simulink model "model"  (R2016a)
settings: Solver=VariableStepAuto  StartTime=0.0  StopTime=30  RelTol=1e-3
values from neighbouring files (symbols this model uses):
  d = 1000    [RobotConstants.mat]
  l0 = 0.16    [RobotConstants.mat]
libraries: simulink x1
settings Model: Creator=Florian  LastModifiedBy=Florian
settings DataIOCC: ExternalInput=[l0]

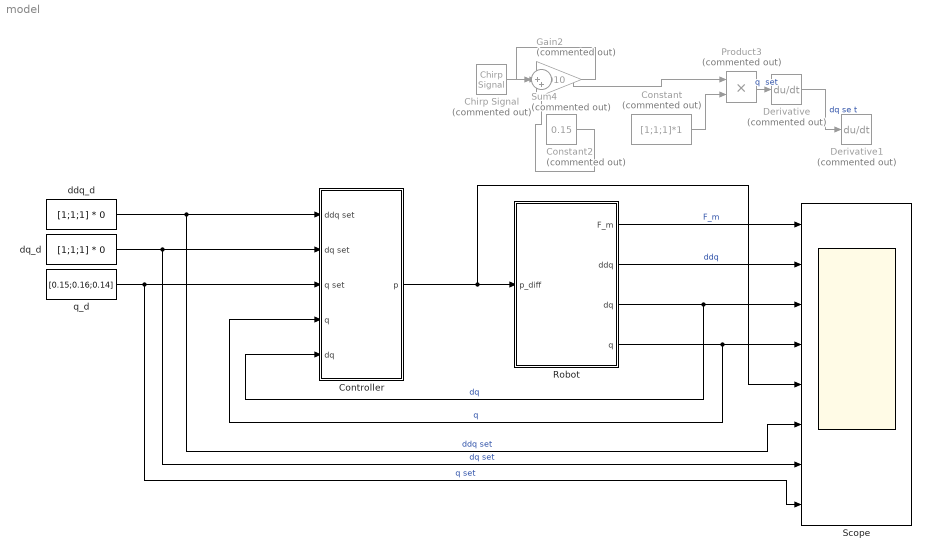
== system model ==
  Chirp Signal : simulink/Sources/Chirp Signal  Commented=on  f1=0.1  T=30  f2=0.1
  Constant : Constant  Commented=on  Value=[1;1;1]*1
  Constant2 : Constant  Commented=on  Value=0.15
  Controller : Subsystem
  Derivative : Derivative  Commented=on
  Derivative1 : Derivative  Commented=on
  Gain2 : Gain  Commented=on  Gain=0.010
  Product3 : Product  Commented=on
  Robot : Subsystem
      mask Display: image('C:\Users\Florian\Documents\Uni\IDP\DVD\Pictures\contibot1seg.JPG');
  Scope : Scope  NumInputPorts=8
  Sum4 : Sum  Commented=on  Inputs=|++
  ddq_d : Constant  Value=[1;1;1] * 0  SampleTime=0.01
  dq_d : Constant  Value=[1;1;1] * 0  SampleTime=0.01
  q_d : Constant  Value=[0.15;0.16;0.14]  SampleTime=0.01
  wires:
  Robot/1(F_m) -> Scope/1  "F_m"
  Robot/2(ddq) -> Scope/2  "ddq"
  Robot/3(dq) -> Controller/5(dq), Scope/3  "dq"
  Robot/4(q) -> Controller/4(q), Scope/4  "q"
  Constant/1 -> Product3/2
  Chirp Signal/1 -> Gain2/1
  Gain2/1 -> Sum4/1
  Sum4/1 -> Product3/1
  Constant2/1 -> Sum4/2
  Product3/1 -> Derivative/1  "q  set"
  Derivative/1 -> Derivative1/1  "dq se t"
  ddq_d/1 -> Controller/1(ddq set), Scope/6  "ddq set"
  Controller/1(p) -> Scope/5, Robot/1(p_diff)
  dq_d/1 -> Scope/7, Controller/2(dq set)  "dq set"
  q_d/1 -> Scope/8, Controller/3(q set)  "q set"

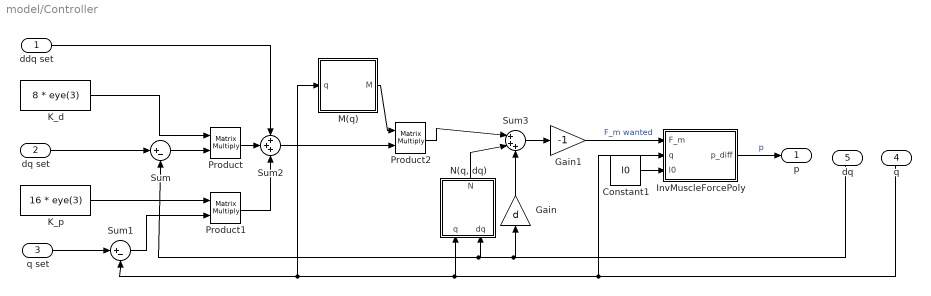
== system model/Controller ==
  ddq set : Inport
  dq set : Inport  Port=2
  q set : Inport  Port=3
  q : Inport  Port=4
  dq : Inport  Port=5
  Constant1 : Constant  Value=l0  SampleTime=0.01
  Gain : Gain  Gain=d
  Gain1 : Gain  Gain=-1
  InvMuscleForcePoly : MATLAB Function  TreatAsAtomicUnit=on
  K_d : Constant  Value=8 * eye(3)  SampleTime=0.01
  K_p : Constant  Value=16 * eye(3)  SampleTime=0.01
  M(q) : MATLAB Function  TreatAsAtomicUnit=on
  "N(q, dq)" : MATLAB Function  TreatAsAtomicUnit=on
  Product : Product  Multiplication=Matrix(*)
  Product1 : Product  Multiplication=Matrix(*)
  Product2 : Product  Multiplication=Matrix(*)
  Sum : Sum  Inputs=|+-
  Sum1 : Sum  Inputs=|+-
  Sum2 : Sum  Inputs=+++
  Sum3 : Sum  Inputs=|+++
  p : Outport
  wires:
  Sum/1 -> Product/2
  M(q)/1(M) -> Product2/1
  Sum2/1 -> Product2/2
  "N(q, dq)"/1(N) -> Sum3/2
  K_p/1 -> Product1/1
  Gain/1 -> Sum3/3
  Sum1/1 -> Product1/2
  Product1/1 -> Sum2/3
  Product2/1 -> Sum3/1
  Product/1 -> Sum2/2
  Sum3/1 -> Gain1/1
  K_d/1 -> Product/1
  Constant1/1 -> InvMuscleForcePoly/3(l0)
  Gain1/1 -> InvMuscleForcePoly/1(F_m)  "F_m wanted"
  InvMuscleForcePoly/1(p_diff) -> p/1  "p"
  dq/1 -> Sum/2, "N(q, dq)"/2(dq), Gain/1
  q set/1 -> Sum1/1
  q/1 -> Sum1/2, M(q)/1(q), "N(q, dq)"/1(q), InvMuscleForcePoly/2(q)
  dq set/1 -> Sum/1
  ddq set/1 -> Sum2/1

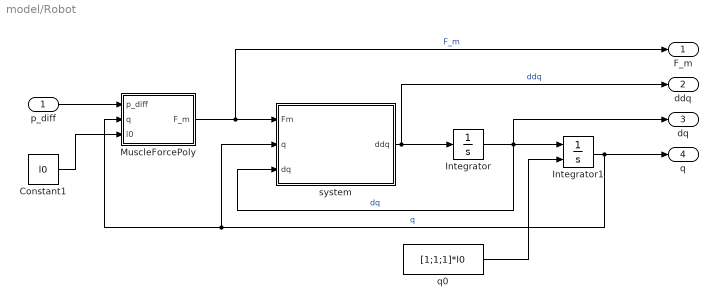
== system model/Robot ==
  p_diff : Inport
  Constant1 : Constant  Value=l0
  Integrator : Integrator  InitialCondition=[1;1;1]*0
  Integrator1 : Integrator  InitialConditionSource=external  InitialCondition=[0.17; 0.15; 0.15]
  MuscleForcePoly : MATLAB Function  TreatAsAtomicUnit=on
  q0 : Constant  Value=[1;1;1]*l0
  system : MATLAB Function  TreatAsAtomicUnit=on
  F_m : Outport
  ddq : Outport  Port=2
  dq : Outport  Port=3
  q : Outport  Port=4
  wires:
  MuscleForcePoly/1(F_m) -> system/1(Fm), F_m/1  "F_m"
  q0/1 -> Integrator1/2
  system/1(ddq) -> ddq/1, Integrator/1  "ddq"
  Integrator1/1 -> q/1, MuscleForcePoly/2(q), system/2(q)  "q"
  Integrator/1 -> dq/1, system/3(dq), Integrator1/1  "dq"
  p_diff/1 -> MuscleForcePoly/1(p_diff)
  Constant1/1 -> MuscleForcePoly/3(l0)

== matlab function model/Robot/MuscleForcePoly ==
  data: p_diff input; F_m output; q input; l0 input
function F_m = fcn(p_diff, q, l0)
%#codegen

%coder.extrinsic('Ffunc');

%p00 = 30.78;
%p10 = 71.9;
%p01 = -22.58;

% p00 = 1.85;
% p10 = 91.44;
% p01 = -28.46;
% p20 = -1.181;
% p11 = -2.827;
% p02 = 1.159;

p00 =       17.64;
p10 =       82.44;
p01 =      -40.53;
p11 =      -2.827;
p02 =       3.249;
p12 =   -0.004285;
p03 =    -0.07887;

h = (l0 - q)/l0 * 100;

F_m = p00 + p10*p_diff + p01*h + p11*p_diff.*h + p02*h.^2 + p12*p_diff.*h.^2 + p03*h.^3 - 17;
%F_m = p00 + p10*p_diff + p01*h + p20*p_diff.^2 + p11*p_diff.*h + p02*h.^2;
%F_m = p00 + p10*p_diff + p01*h;

%F_m = 0 * q;
%F_m = Ffunc(p_diff, q);

== matlab function model/Robot/system ==
  data: Fm input; ddq output; q input; dq input
function ddq = fcn(Fm, q, dq)
%#codegen

%coder.extrinsic('Mfunc');
%coder.extrinsic('Nfunc');

if abs(q(1) - q(2)) < 0.0001 && abs(q(2) - q(3)) < 0.0001
    M = Mfunc2(q);
    N = Nfunc2(q, dq);
    Q = Qfunc2(dq, -Fm);    
else
    M = Mfunc(q);
    N = Nfunc(q, dq);
    Q = Qfunc(dq, -Fm);  
end

c = rcond(M);
if c < 10e-10 || isnan(c)
    M = Mfunc2(q);
    N = Nfunc2(q, dq);
    Q = Qfunc2(dq, -Fm);   
end

invM = inv(M);
ddq = invM * (Q - N);
1+1;

== matlab function model/Controller/M(q) ==
  data: M output; q input
function M = fcn(q)
%#codegen

%coder.extrinsic('Mfunc');
if abs(q(1) - q(2)) < 0.0001 && abs(q(2) - q(3)) < 0.0001
    M = Mfunc2(q);
else
    M = Mfunc(q);
end

== matlab function model/Controller/N(q, dq) ==
  data: N output; q input; dq input
function N = fcn(q, dq)
%#codegen

%coder.extrinsic('Nfunc');
if abs(q(1) - q(2)) < 0.0001 && abs(q(2) - q(3)) < 0.0001
    N = Nfunc2(q, dq);
else
    N = Nfunc(q, dq);
end

== matlab function model/Controller/InvMuscleForcePoly ==
  data: F_m input; p_diff output; q input; l0 input
function p_diff = fcn(F_m, q, l0)
%#codegen

% coder.extrinsic('Pfunc');
% 
% p00 = 30.78; %1.85;
% p10 = 71.9;%91.44;
% p01 = -22.58;%-28.46;
% %p20 = -1.181;
% %p11 = -2.827;
% %p02 = 1.159;
% 
% h = (l0 - q)/l0 * 100;
% 
% p_diff = (F_m - p00 - p01*h) / p10;

%wurzel = sqrt((p10 + p11*h).^2 - 4 * p20 * (p00 + p01*h + p02*h.^2 - F_m));
%p_diff1 = (-p10-p11*h + wurzel)/(2*p20);
%p_diff2 = (-p10-p11*h - wurzel)/(2*p20);

%p_diff = max(p_diff1, p_diff2);

%p_diff = 0 * F_m;
%p_diff = Pfunc(F_m, q);

p00 =       17.64;
p10 =       82.44;
p01 =      -40.53;
p11 =      -2.827;
p02 =       3.249;
p12 =   -0.004285;
p03 =    -0.07887;

h = (l0 - q)/l0 * 100;

p_diff = (F_m - p00 - p01 * h - p02 * h.^2 - p03 * h.^3 + 17) ./ (p10 + p11 * h + p12 * h.^2);

for i = 1:length(p_diff)
    if p_diff(i) < 0
        p_diff(i) = 0;
    elseif p_diff(i) > 6
        p_diff(i) = 6;
    end
end
